simulink model "robot_control_simulink_draft"  (R2022a)
settings: Solver=VariableStepAuto  StartTime=0.0  StopTime=10.0  RelTol=1e-3
libraries: matrix_library x2, simulink x2
settings Model: Creator=kvasios  LastModifiedBy=kvasios

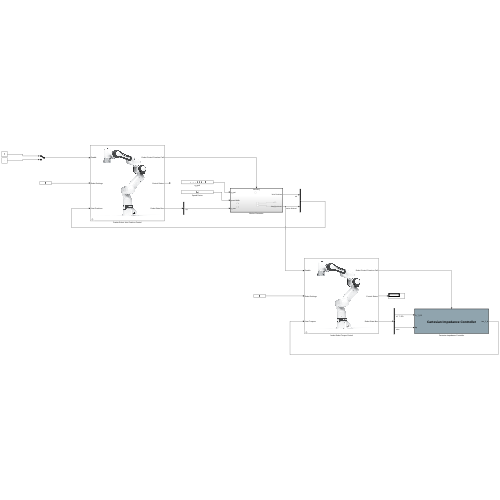
[thumbnail: Simulink's stored preview of the top-level diagram]
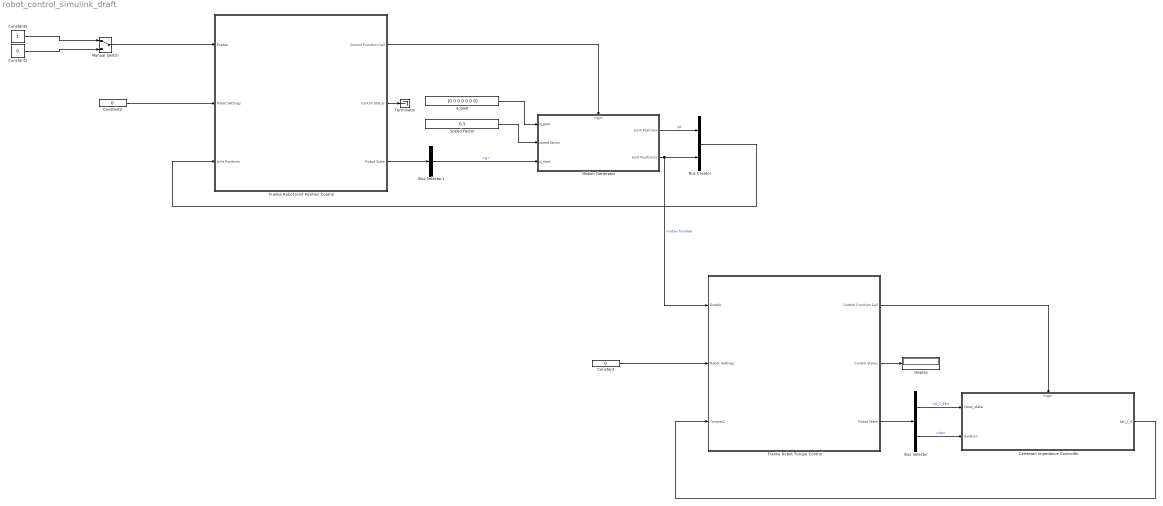
== system robot_control_simulink_draft ==
  Bus Creator : BusCreator  Inputs=2
  Bus Selector : BusSelector  OutputSignals=O_T_EE,dq
  Bus Selector1 : BusSelector  OutputSignals=q
  Cartesian Impedance Controller : Subsystem
      mask Display:
      | disp('{\bf\fontsize{18}Cartesian Impedance Controller}', 'texmode','on');
      | 
      | block_icon('Controller')
      | 
      | port_label('output',1,'tau_J_d');
      | 
      | port_label('input',1,'O_T_EE');
      | port_label('input',2,'dq');
  Constant : Constant  Value=0
  Constant1 : Constant  Value=0
  Constant2 : Constant
  Constant3 : Constant  Value=0
  Display : Display
  Franka Robot Joint Position Control : Subsystem
      mask Display:
      | image(fullfile(franka_toolbox_installation_path_get(),'data','images','franka_robot_no_ee.png'));
      | 
      | port_label('input',1,'Enable');
      | port_label('input',2,'Robot Settings');
      | port_label('input',3,'Joint Positions');
      | port_label('output',1,'Robot Control Function Call');
      | port_label('output',2,'Control Status');
      | port_label('output',3,'Robot State Bus');
      | 
      | % gripper_attached_flag = 0;
      | %
      | % gripper_selection = get_param(gcb,'gripper_selection');
      | %
      | % if strcmp(gripper_selection,'Franka Gripper')
      | %     gripper_attached_flag = 1;
      | %     port_label('input',1,'gripper_control');
      | % end
      | %
      | % if strcmp(gripper_selection,'Franka Vacuum Gripper')
      | %     gripper_attached_flag = 1;
      | %     port_label('input',1,'vacuum_gripper_control');
      | % end
      | %
      | % control_mode = get_param(gcb,'control_mode');
      | %
      | % elbow_control = get_param(gcb,'elbow_control');
      | %
      | % switch control_mode
      | %    case 'Torque Control'
      | %       port_label('input',1+gripper_attached_flag,'tau_J_d');
      | %    case 'Torque Control - Joint Positions'
      | %       port_label('input',1+gripper_attached_flag,'q_d');
      | %       port_label('input',2+gripper_attached_flag,'tau_J_d');
      | %    case 'Torque Control - Joint Velocities'
      | %       port_label('input',1+gripper_attached_flag,'dq_d');
      | %       port_label('input',2+gripper_attached_flag,'tau_J_d');
      | %    case 'Torque Control - Cartesian Pose'
      | %       port_label('input',1+gripper_attached_flag,'O_T_EE_d');
      | %       if strcmp(elbow_control, 'on')
      | %         port_label('input',2+gripper_attached_flag,'elbow_d');
      | %         port_label('input',3+gripper_attached_flag,'tau_J_d');
      | %       else
      | %         port_label('input',2+gripper_attached_flag,'tau_J_d');
      | %       end
      | %     case 'Torque Control - Cartesian Velocities'
      | %       port_label('input',1+gripper_attached_flag,'O_dP_EE_d');
      | %       if strcmp(elbow_control, 'on')
      | %         port_label('input',2+gripper_attached_flag,'elbow_d');
      | %         port_label('input',3+gripper_attached_flag,'tau_J_d');
      | %       else
      | %         port_label('input',2+gripper_attached_flag,'tau_J_d');
      | %       end
      | %     case 'Joint Positions - Internal Controller Mode'
      | %       port_label('input',1+gripper_attached_flag,'q_d');
      | %     case 'Joint Velocities - Internal Controller Mode'
      | %       port_label('input',1+gripper_attached_flag,'dq_d');
      | %     case 'Cartesian Pose - Internal Controller Mode'
      | %       port_label('input',1+gripper_attached_flag,'O_T_EE_d');
      | %       if strcmp(elbow_control, 'on')
      | %         port_label('input',2+gripper_attached_flag,'elbow_d');
      | %       end
      | %     case 'Cartesian Velocities - Internal Controller Mode'
      | %       port_label('input',1+gripper_attached_flag,'O_dP_EE_d');
      | %       if strcmp(elbow_control, 'on')
      | %         port_label('input',2+gripper_attached_flag,'elbow_d');
      | %       end
      | % end
      | 
      | % img_x = 230;
      | % img_y = 250;
      | %
      | % img_length = 50;
      | % img_height = 50;
      | %
      | % block_length_lib = 295;
      | % block_height_lib = 316;
      | %
      | % position = get_param(gcb, 'position');
      | %
      | % block_length = abs(position(1) - position(3));
      | % block_height = abs(position(2) - position(4));
      | %
      | % imagePath = fullfile(franka_toolbox_installation_path_get,'data','images','franka_emika_logo.png');
      | % pic=imread(imagePath);
      | % image(pic, [ abs(img_x + (block_length - block_length_lib)) abs(img_y + (block_height - block_height_lib)) img_length img_height ]);
      | %
      | % color('black');
      | % text(258 + (block_length - 295), 163 + (block_height - 250), 'Franka\nRobot Control', 'horizontalAlignment', 'center');
  Franka Robot Torque Control : Subsystem
      mask Display:
      | image(fullfile(franka_toolbox_installation_path_get(),'data','images','franka_robot_no_ee.png'));
      | 
      | port_label('input',1,'Enable');
      | port_label('input',2,'Robot Settings');
      | port_label('input',3,'Joint Torques');
      | port_label('output',1,'Robot Control Function Call');
      | port_label('output',2,'Control Status');
      | port_label('output',3,'Robot State Bus');
      | 
      | % gripper_attached_flag = 0;
      | %
      | % gripper_selection = get_param(gcb,'gripper_selection');
      | %
      | % if strcmp(gripper_selection,'Franka Gripper')
      | %     gripper_attached_flag = 1;
      | %     port_label('input',1,'gripper_control');
      | % end
      | %
      | % if strcmp(gripper_selection,'Franka Vacuum Gripper')
      | %     gripper_attached_flag = 1;
      | %     port_label('input',1,'vacuum_gripper_control');
      | % end
      | %
      | % control_mode = get_param(gcb,'control_mode');
      | %
      | % elbow_control = get_param(gcb,'elbow_control');
      | %
      | % switch control_mode
      | %    case 'Torque Control'
      | %       port_label('input',1+gripper_attached_flag,'tau_J_d');
      | %    case 'Torque Control - Joint Positions'
      | %       port_label('input',1+gripper_attached_flag,'q_d');
      | %       port_label('input',2+gripper_attached_flag,'tau_J_d');
      | %    case 'Torque Control - Joint Velocities'
      | %       port_label('input',1+gripper_attached_flag,'dq_d');
      | %       port_label('input',2+gripper_attached_flag,'tau_J_d');
      | %    case 'Torque Control - Cartesian Pose'
      | %       port_label('input',1+gripper_attached_flag,'O_T_EE_d');
      | %       if strcmp(elbow_control, 'on')
      | %         port_label('input',2+gripper_attached_flag,'elbow_d');
      | %         port_label('input',3+gripper_attached_flag,'tau_J_d');
      | %       else
      | %         port_label('input',2+gripper_attached_flag,'tau_J_d');
      | %       end
      | %     case 'Torque Control - Cartesian Velocities'
      | %       port_label('input',1+gripper_attached_flag,'O_dP_EE_d');
      | %       if strcmp(elbow_control, 'on')
      | %         port_label('input',2+gripper_attached_flag,'elbow_d');
      | %         port_label('input',3+gripper_attached_flag,'tau_J_d');
      | %       else
      | %         port_label('input',2+gripper_attached_flag,'tau_J_d');
      | %       end
      | %     case 'Joint Positions - Internal Controller Mode'
      | %       port_label('input',1+gripper_attached_flag,'q_d');
      | %     case 'Joint Velocities - Internal Controller Mode'
      | %       port_label('input',1+gripper_attached_flag,'dq_d');
      | %     case 'Cartesian Pose - Internal Controller Mode'
      | %       port_label('input',1+gripper_attached_flag,'O_T_EE_d');
      | %       if strcmp(elbow_control, 'on')
      | %         port_label('input',2+gripper_attached_flag,'elbow_d');
      | %       end
      | %     case 'Cartesian Velocities - Internal Controller Mode'
      | %       port_label('input',1+gripper_attached_flag,'O_dP_EE_d');
      | %       if strcmp(elbow_control, 'on')
      | %         port_label('input',2+gripper_attached_flag,'elbow_d');
      | %       end
      | % end
      | 
      | % img_x = 230;
      | % img_y = 250;
      | %
      | % img_length = 50;
      | % img_height = 50;
      | %
      | % block_length_lib = 295;
      | % block_height_lib = 316;
      | %
      | % position = get_param(gcb, 'position');
      | %
      | % block_length = abs(position(1) - position(3));
      | % block_height = abs(position(2) - position(4));
      | %
      | % imagePath = fullfile(franka_toolbox_installation_path_get,'data','images','franka_emika_logo.png');
      | % pic=imread(imagePath);
      | % image(pic, [ abs(img_x + (block_length - block_length_lib)) abs(img_y + (block_height - block_height_lib)) img_length img_height ]);
      | %
      | % color('black');
      | % text(258 + (block_length - 295), 163 + (block_height - 250), 'Franka\nRobot Control', 'horizontalAlignment', 'center');
  Manual Switch : ManualSwitch
  Motion Generator : Subsystem
  Speed Factor : Constant  Value=0.5
  Terminator : Terminator
  q_goal : Constant  Value=[0 0 0 0 0 0 0]
  wires:
  Franka Robot Torque Control/1(Control Function Call) -> Cartesian Impedance Controller/Trigger
  Bus Selector/1 -> Cartesian Impedance Controller/1(robot_state)  "<O_T_EE>"
  Bus Selector/2 -> Cartesian Impedance Controller/2(duration)  "<dq>"
  Franka Robot Torque Control/3(Robot State) -> Bus Selector/1
  Cartesian Impedance Controller/1(tau_J_d) -> Franka Robot Torque Control/3(Torques2)
  Constant/1 -> Franka Robot Torque Control/2(Robot Settings)
  Franka Robot Torque Control/2(Control Status) -> Display/1
  q_goal/1 -> Motion Generator/1(q_goal)
  Speed Factor/1 -> Motion Generator/2(speed factor)
  Franka Robot Joint Position Control/3(Robot State) -> Bus Selector1/1
  Bus Selector1/1 -> Motion Generator/3(q_start)  "<q>"
  Franka Robot Joint Position Control/1(Control Function Call) -> Motion Generator/Trigger
  Bus Creator/1 -> Franka Robot Joint Position Control/3(Joint Positions)
  Motion Generator/1(Joint Positions) -> Bus Creator/1  "qd"
  Motion Generator/2(Joint Positions1) -> Bus Creator/2, Franka Robot Torque Control/1(Enable)  "motion finished"
  Franka Robot Joint Position Control/2(Control Status) -> Terminator/1
  Manual Switch/1 -> Franka Robot Joint Position Control/1(Enable)
  Constant2/1 -> Manual Switch/1
  Constant1/1 -> Manual Switch/2
  Constant3/1 -> Franka Robot Joint Position Control/2(Robot Settings)

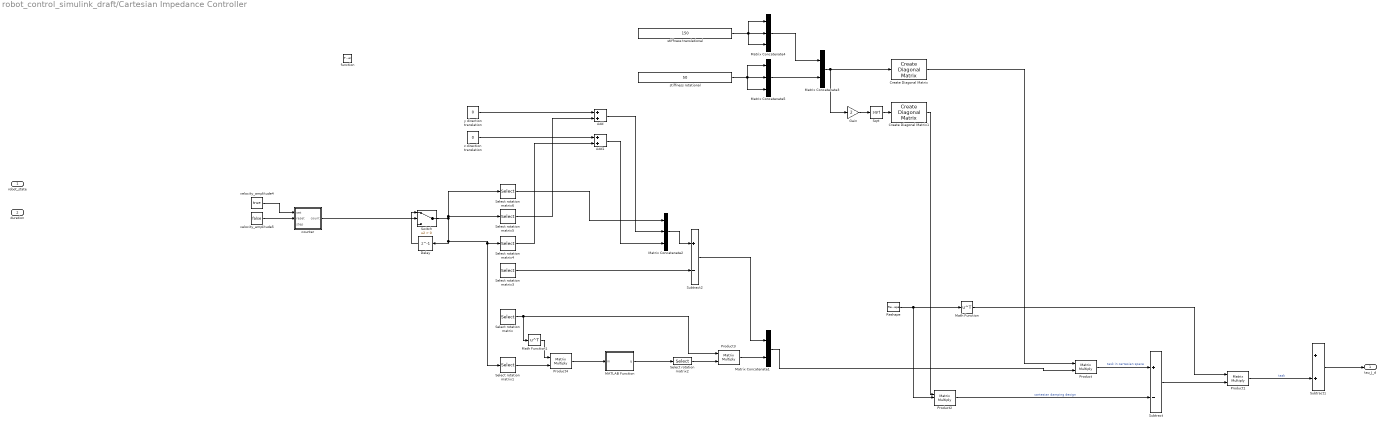
== system robot_control_simulink_draft/Cartesian Impedance Controller ==
  robot_state : Inport
  duration : Inport  Port=2
  function : TriggerPort  TriggerType=function-call  VariantControl=(inherit)  StatesWhenEnabling=reset
  Add : Sum
  Add1 : Sum
  Create Diagonal Matrix : matrix_library/Create Diagonal Matrix
      settings: SourceProductBaseCode=SL
  Create Diagonal Matrix1 : matrix_library/Create Diagonal Matrix
      settings: SourceProductBaseCode=SL
  Delay : Delay  DelayLength=1
  Gain : Gain  Gain=2
  MATLAB Function : MATLAB Function  TreatAsAtomicUnit=on
  Math Function : Math  Operator=transpose  SignedPower=on
  Math Function1 : Math  Operator=transpose  SignedPower=on
  Matrix Concatenate1 : Concatenate
  Matrix Concatenate2 : Concatenate  NumInputs=3
  Matrix Concatenate3 : Concatenate
  Matrix Concatenate4 : Concatenate  NumInputs=3
  Matrix Concatenate5 : Concatenate  NumInputs=3
  Product{,1,3..4} (4 alike) : Product  Multiplication=Matrix(*)
  Product2 : Product  Inputs=3  Multiplication=Matrix(*)
  Reshape : Reshape  OutputDimensionality=Customize  OutputDimensions=[6,7]
  Select rotation matrix : Selector  NumberOfDimensions=2  InputPortWidth=3  IndexOptions=Index vector (dialog),Index vector (dialog)  Indices=[1,2,3],[1 2 3]  OutputSizes=1
  Select rotation matrix1 : Selector  NumberOfDimensions=2  InputPortWidth=3  IndexOptions=Index vector (dialog),Index vector (dialog)  Indices=[1,2,3],[1 2 3]  OutputSizes=1
  Select rotation matrix2 : Selector  InputPortWidth=4  IndexOptions=Index vector (dialog)  Indices=[2,3,4]  OutputSizes=1
  Select rotation matrix3 : Selector  NumberOfDimensions=2  InputPortWidth=3  IndexOptions=Index vector (dialog),Index vector (dialog)  Indices=[1,2,3],[4]  OutputSizes=1
  Select rotation matrix4 : Selector  NumberOfDimensions=2  InputPortWidth=3  IndexOptions=Index vector (dialog),Index vector (dialog)  Indices=[3],[4]  OutputSizes=1
  Select rotation matrix5 : Selector  NumberOfDimensions=2  InputPortWidth=3  IndexOptions=Index vector (dialog),Index vector (dialog)  Indices=[2],[4]  OutputSizes=1
  Select rotation matrix6 : Selector  NumberOfDimensions=2  InputPortWidth=3  IndexOptions=Index vector (dialog),Index vector (dialog)  Indices=[1],[4]  OutputSizes=1
  Sqrt : Sqrt
  Subtract : Sum  Inputs=+-
  Subtract1 : Sum
  Subtract2 : Sum  Inputs=+-
  Switch : Switch  Criteria=u2 > Threshold  SaturateOnIntegerOverflow=off  InputSameDT=off
  counter : Subsystem
  stiffness rotational : Constant  Value=50  VectorParams1D=off
  stiffness translational : Constant  Value=150  VectorParams1D=off
  velocity_amplitude4 : Constant  Value=true  VectorParams1D=off
  velocity_amplitude5 : Constant  Value=false  VectorParams1D=off
  y direction translation : Constant  Value=0
  z direction translation : Constant  Value=0
  tau_J_d : Outport  VectorParamsAs1DForOutWhenUnconnected=off
  wires:
  stiffness rotational/1 -> Matrix Concatenate5/2, Matrix Concatenate5/1, Matrix Concatenate5/3
  Matrix Concatenate5/1 -> Matrix Concatenate3/2
  Matrix Concatenate4/1 -> Matrix Concatenate3/1
  stiffness translational/1 -> Matrix Concatenate4/2, Matrix Concatenate4/3, Matrix Concatenate4/1
  Create Diagonal Matrix/1 -> Product/1
  Sqrt/1 -> Create Diagonal Matrix1/1
  Gain/1 -> Sqrt/1
  Matrix Concatenate3/1 -> Create Diagonal Matrix/1, Gain/1
  Add1/1 -> Matrix Concatenate2/3
  Select rotation matrix4/1 -> Add1/2
  z direction translation/1 -> Add1/1
  Add/1 -> Matrix Concatenate2/2
  Select rotation matrix5/1 -> Add/2
  y direction translation/1 -> Add/1
  Select rotation matrix6/1 -> Matrix Concatenate2/1
  Matrix Concatenate2/1 -> Subtract2/1
  ? -> counter/3(step)
  velocity_amplitude5/1 -> counter/2(reset)
  counter/1(count) -> Switch/2
  velocity_amplitude4/1 -> counter/1(set)
  Delay/1 -> Switch/1
  Math Function1/1 -> Product4/1
  Select rotation matrix1/1 -> Product4/2
  Product3/1 -> Matrix Concatenate1/2
  Select rotation matrix/1 -> Product3/1, Math Function1/1
  Matrix Concatenate1/1 -> Product/2
  Select rotation matrix2/1 -> Product3/2
  Subtract/1 -> Product1/2
  Product4/1 -> MATLAB Function/1(m)
  MATLAB Function/1(q) -> Select rotation matrix2/1
  Subtract2/1 -> Matrix Concatenate1/1
  Select rotation matrix3/1 -> Subtract2/2
  Switch/1 -> Select rotation matrix1/1, Select rotation matrix4/1, Delay/1, Select rotation matrix5/1, Select rotation matrix6/1
  ? -> Switch/3, Select rotation matrix/1, Select rotation matrix3/1
  Product1/1 -> Subtract1/2  "task"
  Subtract1/1 -> tau_J_d/1
  Create Diagonal Matrix1/1 -> Product2/1
  ? -> Product2/3
  ? -> Subtract1/1  "coriolis"
  Product2/1 -> Subtract/2  "cartesian damping design"
  Product/1 -> Subtract/1  "task in cartesian space"
  Math Function/1 -> Product1/1
  Reshape/1 -> Math Function/1, Product2/2
  ? -> Reshape/1

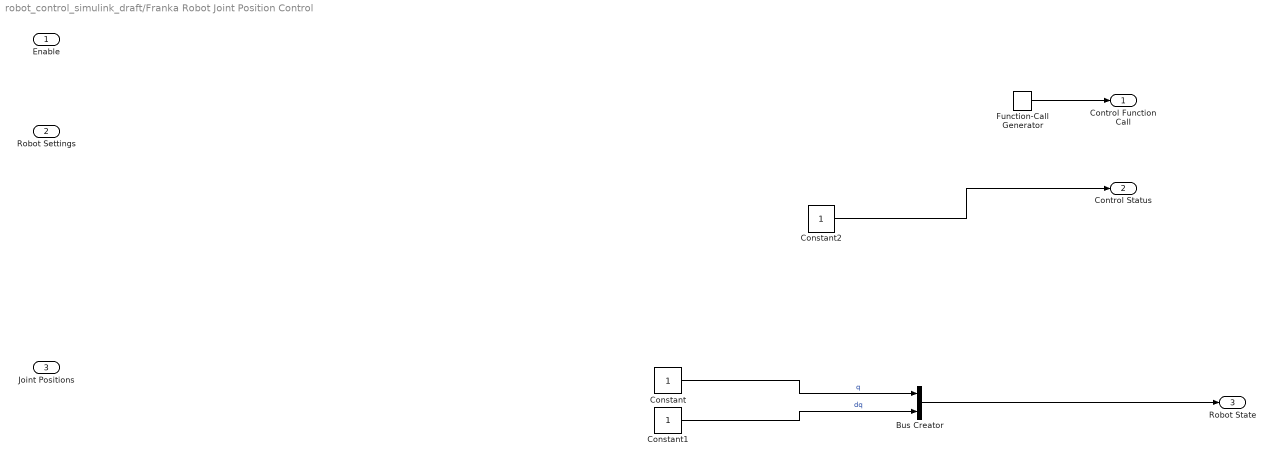
== system robot_control_simulink_draft/Franka Robot Joint Position Control ==
  Enable : Inport
  Robot Settings : Inport  Port=2
  Joint Positions : Inport  Port=3
  Bus Creator : BusCreator  Inputs=2
  Constant : Constant
  Constant1 : Constant
  Constant2 : Constant
  Function-Call Generator : simulink/Ports & Subsystems/Function-Call Generator  sample_time=1  numberOfIterations=1  DisallowWideOutput=off
  Control Function Call : Outport
  Control Status : Outport  Port=2
  Robot State : Outport  Port=3
  wires:
  Constant2/1 -> Control Status/1
  Constant1/1 -> Bus Creator/2  "dq"
  Constant/1 -> Bus Creator/1  "q"
  Bus Creator/1 -> Robot State/1
  Function-Call Generator/1 -> Control Function Call/1

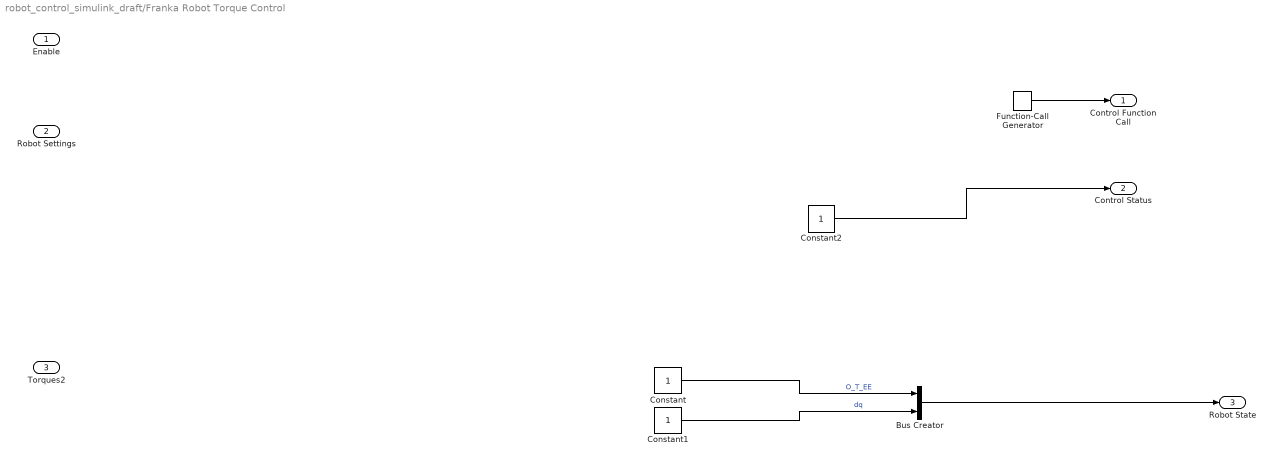
== system robot_control_simulink_draft/Franka Robot Torque Control ==
  Enable : Inport
  Robot Settings : Inport  Port=2
  Torques2 : Inport  Port=3
  Bus Creator : BusCreator  Inputs=2
  Constant : Constant
  Constant1 : Constant
  Constant2 : Constant
  Function-Call Generator : simulink/Ports & Subsystems/Function-Call Generator  sample_time=1  numberOfIterations=1  DisallowWideOutput=off
  Control Function Call : Outport
  Control Status : Outport  Port=2
  Robot State : Outport  Port=3
  wires:
  Function-Call Generator/1 -> Control Function Call/1
  Bus Creator/1 -> Robot State/1
  Constant/1 -> Bus Creator/1  "O_T_EE"
  Constant1/1 -> Bus Creator/2  "dq"
  Constant2/1 -> Control Status/1

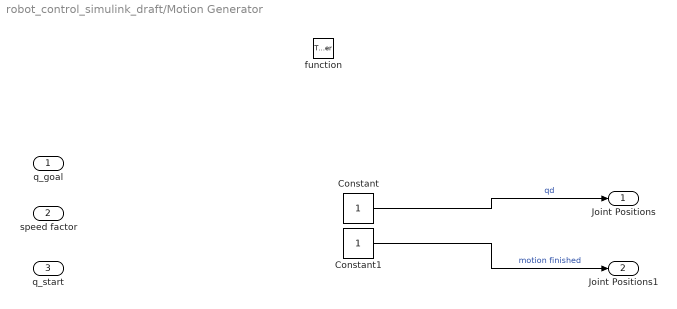
== system robot_control_simulink_draft/Motion Generator ==
  q_goal : Inport
  speed factor : Inport  Port=2
  q_start : Inport  Port=3
  function : TriggerPort  TriggerType=function-call  VariantControl=(inherit)  StatesWhenEnabling=reset
  Constant : Constant
  Constant1 : Constant
  Joint Positions : Outport
  Joint Positions1 : Outport  Port=2
  wires:
  Constant/1 -> Joint Positions/1  "qd"
  Constant1/1 -> Joint Positions1/1  "motion finished"

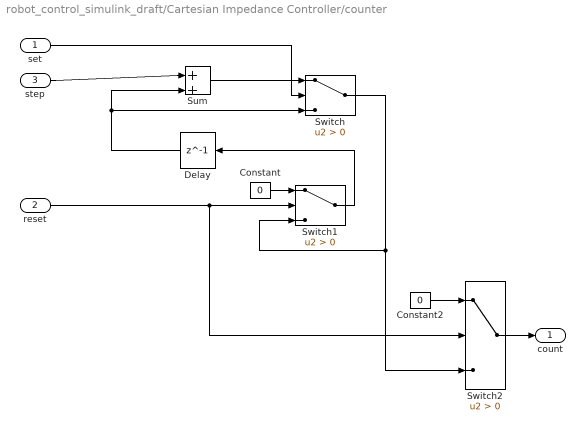
== system robot_control_simulink_draft/Cartesian Impedance Controller/counter ==
  set : Inport  OutDataTypeStr=boolean
  reset : Inport  Port=2  OutDataTypeStr=boolean
  step : Inport  Port=3  OutDataTypeStr=double
  Constant : Constant  Value=0  OutDataTypeStr=double
  Constant2 : Constant  Value=0  OutDataTypeStr=double
  Delay : Delay  DelayLength=1  InitialCondition=0
  Sum : Sum  Inputs=|++
  Switch : Switch  Criteria=u2 > Threshold  SaturateOnIntegerOverflow=off  InputSameDT=off
  Switch1 : Switch  Criteria=u2 > Threshold  OutDataTypeStr=double  SaturateOnIntegerOverflow=off  InputSameDT=off
  Switch2 : Switch  Criteria=u2 > Threshold  OutDataTypeStr=double  SaturateOnIntegerOverflow=off  InputSameDT=off
  count : Outport  OutDataTypeStr=double  VectorParamsAs1DForOutWhenUnconnected=off
  wires:
  Switch1/1 -> Delay/1
  Constant/1 -> Switch1/1
  reset/1 -> Switch2/2, Switch1/2
  Delay/1 -> Switch/3, Sum/2
  step/1 -> Sum/1
  Switch/1 -> Switch2/3, Switch1/3
  set/1 -> Switch/2
  Sum/1 -> Switch/1
  Constant2/1 -> Switch2/1
  Switch2/1 -> count/1

== matlab function robot_control_simulink_draft/Cartesian Impedance Controller/MATLAB Function ==
  data: m input; q output
function q = rotm2quat(m)

m00 = m(1,1);
m01 = m(1,2);
m02 = m(1,3);

m10 = m(2,1);
m11 = m(2,2);
m12 = m(2,3);

m20 = m(3,1);
m21 = m(3,2);
m22 = m(3,3);

tr = m00 + m11 + m22;

if (tr > 0) 
  S = sqrt(tr+1.0) * 2; % S=4*qw 
  qw = 0.25 * S;
  qx = (m21 - m12) / S;
  qy = (m02 - m20) / S; 
  qz = (m10 - m01) / S; 
elseif ((m00 > m11) && (m00 > m22))
  S = sqrt(1.0 + m00 - m11 - m22) * 2;  %S=4*qx 
  qw = (m21 - m12) / S;
  qx = 0.25 * S;
  qy = (m01 + m10) / S; 
  qz = (m02 + m20) / S; 
elseif (m11 > m22) 
  S = sqrt(1.0 + m11 - m00 - m22) * 2; % S=4*qy
  qw = (m02 - m20) / S;
  qx = (m01 + m10) / S; 
  qy = 0.25 * S;
  qz = (m12 + m21) / S; 
else 
  S = sqrt(1.0 + m22 - m00 - m11) * 2; % S=4*qz
  qw = (m10 - m01) / S;
  qx = (m02 + m20) / S;
  qy = (m12 + m21) / S;
  qz = 0.25 * S;
end

q = [qw,qx,qy,qz]';
